simulink model "SimulateurNL_AERO_Cmd_LQI"  (R2023b)
settings: Solver=ode23tb  StartTime=0.0  StopTime=25  RelTol=1e-3
values from neighbouring files (symbols this model uses):
  Dm = 0.0071    [InitCommande_Aero.m]
  Dt = 0.158    [InitCommande_Aero.m]
  F0_h = Mb*g*Dm/Dt*sin(theta_h*pi/180)    [InitCommande_Aero.m]
  g = 9.81    [InitCommande_Aero.m]
  K_lqi = lqr(Aa, B1a, Q, R)    [InitCommande_Aero.m]
  Kw = Ka(1)    [InitCommande_Aero.m]    (also in matlab_variables_2_2.mat = 0.240350108962)
  Kz = Ka(2)    [InitCommande_Aero.m]    (also in matlab_variables_2_2.mat = 4.57892915652)
  Mb = 1.15    [InitCommande_Aero.m]
  omega_h = [-250 -200 -150 150 200 250]    [InitCommande_Aero.m]
  Te1 = 0.002    [InitCommande_Aero.m]    (also in apoio.m = 0.0005; matlab_variables_2_2.mat)
  Te2 = 0.02    [InitCommande_Aero.m]
libraries: simulink_extras x1
settings Model: Creator=Stagiaire  LastModifiedBy=rick
settings SolverCC: AlgebraicLoopSolver=TrustRegion
settings DataIOCC: ReturnWorkspaceOutputs=off
settings OptimizationCC: ReuseModelBlockBuffer=off
settings DebuggingCC: UnconnectedInputMsg=warning  UnconnectedOutputMsg=warning  UnconnectedLineMsg=warning  ArithmeticOperatorsInVariantConditions=warning
settings ModelReferenceCC: EnableRefExpFcnMdlSchedulingChecks=on
settings SFSimCC: CustomCodeUndefinedFunction=UseInterfaceOnly

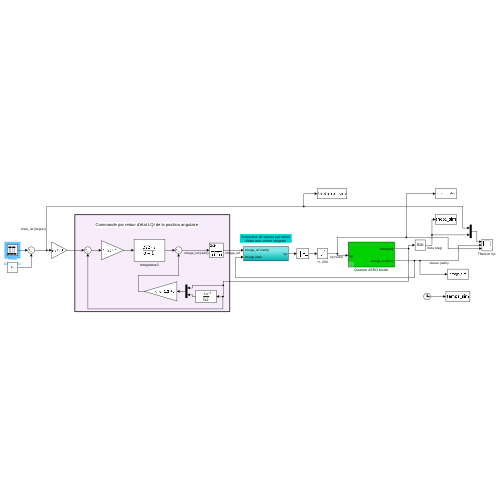
[thumbnail: Simulink's stored preview of the top-level diagram]
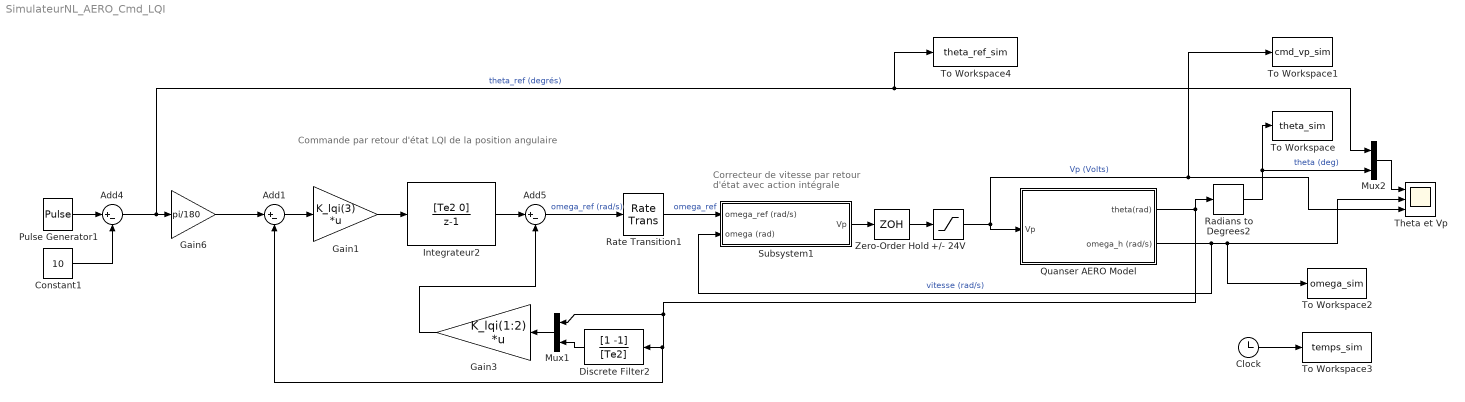
== system SimulateurNL_AERO_Cmd_LQI ==
  note: Correcteur de vitesse par retour d'état avec action intégrale
  note: Commande par retour d'état LQI de la position angulaire
  +/- 24V : Saturate  UpperLimit=24  LowerLimit=-24
  Add1 : Sum  Inputs=|+-
  Add4 : Sum  Inputs=|+-
  Add5 : Sum  Inputs=|+-
  Clock : Clock
  Constant1 : Constant  Value=10
  Discrete Filter2 : DiscreteFilter  Numerator=[1 -1]  Denominator=[Te2]  SampleTime=Te2
  Gain1 : Gain  Gain=K_lqi(3)  Multiplication=Matrix(K*u)
  Gain3 : Gain  Gain=K_lqi(1:2)  Multiplication=Matrix(K*u)
  Gain6 : Gain  Gain=pi/180
  Integrateur2 : DiscreteTransferFcn  Numerator=[Te2 0]  Denominator=[1 -1]  SampleTime=Te2
  Mux1 : Mux  Inputs=2
  Mux2 : Mux  Inputs=2
  Pulse Generator1 : DiscretePulseGenerator  Amplitude=20  Period=ceil(20/Te2)  PulseWidth=ceil(10/Te2)  SampleTime=Te2
  Quanser AERO Model : Subsystem  mask{Kv=19.66, tau=0.18, Jp=0.046, Dp=0.0091, F0_table=F0_h, W_table=omega_h}
  Radians to Degrees2 : simulink_extras/Transformations/Radians to Degrees
  Rate Transition1 : RateTransition  OutPortSampleTime=Te1
  Subsystem1 : Subsystem
  "Theta et Vp " : Scope  NumInputPorts=3
  To Workspace : ToWorkspace  VariableName=theta_sim  SampleTime=-1
      settings: Decimation=10  Save2DSignal=2-D array (concatenate along first dimension)
  To Workspace1 : ToWorkspace  VariableName=cmd_vp_sim  SampleTime=-1
      settings: Decimation=10  Save2DSignal=2-D array (concatenate along first dimension)
  To Workspace2 : ToWorkspace  VariableName=omega_sim  SampleTime=-1
      settings: Decimation=10  Save2DSignal=2-D array (concatenate along first dimension)
  To Workspace3 : ToWorkspace  VariableName=temps_sim  SampleTime=-1
      settings: Decimation=10  Save2DSignal=2-D array (concatenate along first dimension)
  To Workspace4 : ToWorkspace  VariableName=theta_ref_sim  SampleTime=-1
      settings: Decimation=10  Save2DSignal=2-D array (concatenate along first dimension)
  Zero-Order Hold : ZeroOrderHold  SampleTime=Te1
  wires:
  +/- 24V/1 -> To Workspace1/1, "Theta et Vp "/3, Quanser AERO Model/1(Vp)  "Vp (Volts)"
  Quanser AERO Model/2(omega_h (rad/s)) -> Subsystem1/2(omega (rad)), To Workspace2/1, "Theta et Vp "/2  "vitesse (rad/s)"
  Quanser AERO Model/1(theta(rad)) -> Radians to Degrees2/1, Add1/2, Discrete Filter2/1, Mux1/1
  Zero-Order Hold/1 -> +/- 24V/1
  Rate Transition1/1 -> Subsystem1/1(omega_ref (rad/s))  "omega_ref"
  Gain3/1 -> Add5/2
  Add5/1 -> Rate Transition1/1  "omega_ref (rad/s)"
  Mux1/1 -> Gain3/1
  Add4/1 -> To Workspace4/1, Mux2/1, Gain6/1  "theta_ref (degrés)"
  Pulse Generator1/1 -> Add4/1
  Constant1/1 -> Add4/2
  Subsystem1/1(Vp) -> Zero-Order Hold/1
  Mux2/1 -> "Theta et Vp "/1
  Radians to Degrees2/1 -> To Workspace/1, Mux2/2  "theta (deg)"
  Discrete Filter2/1 -> Mux1/2
  Gain1/1 -> Integrateur2/1
  Integrateur2/1 -> Add5/1
  Gain6/1 -> Add1/1
  Add1/1 -> Gain1/1
  Clock/1 -> To Workspace3/1

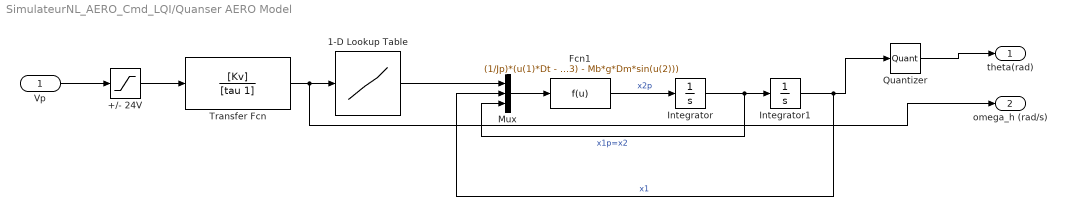
== system SimulateurNL_AERO_Cmd_LQI/Quanser AERO Model ==
  Vp : Inport
  +/- 24V : Saturate  UpperLimit=24  LowerLimit=-24
  1-D Lookup Table : Lookup_n-D  NumberOfTableDimensions=1  BreakpointsForDimension1=W_table  Table=F0_table  InternalRulePriority=Speed  RndMeth=Simplest
  Fcn1 : Fcn  Expr=(1/Jp)*(u(1)*Dt - Dp*u(3) - Mb*g*Dm*sin(u(2)))
  Integrator : Integrator
  Integrator1 : Integrator
  Mux : Mux  Inputs=3
  Quantizer : Quantizer  QuantizationInterval=2*pi/2048
  Transfer Fcn : TransferFcn  Numerator=[Kv]  Denominator=[tau 1]
  theta(rad) : Outport  VectorParamsAs1DForOutWhenUnconnected=off
  omega_h (rad/s) : Outport  Port=2  VectorParamsAs1DForOutWhenUnconnected=off
  wires:
  1-D Lookup Table/1 -> Mux/1
  Mux/1 -> Fcn1/1
  Integrator/1 -> Integrator1/1, Mux/3  "x1p=x2"
  Fcn1/1 -> Integrator/1  "x2p"
  Transfer Fcn/1 -> omega_h (rad/s)/1, 1-D Lookup Table/1
  Quantizer/1 -> theta(rad)/1
  Vp/1 -> +/- 24V/1
  Integrator1/1 -> Quantizer/1, Mux/2  "x1"
  +/- 24V/1 -> Transfer Fcn/1

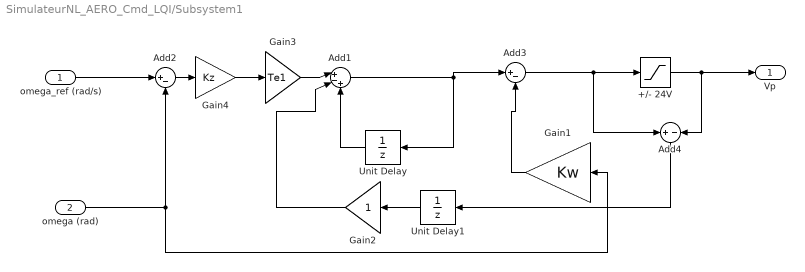
== system SimulateurNL_AERO_Cmd_LQI/Subsystem1 ==
  omega_ref (rad/s) : Inport
  omega (rad) : Inport  Port=2
  +/- 24V : Saturate  UpperLimit=24  LowerLimit=-24
  Add1 : Sum  Inputs=|+-+
  Add2 : Sum  Inputs=|+-
  Add3 : Sum  Inputs=|+-
  Add4 : Sum  Inputs=+-
  Gain1 : Gain  Gain=Kw
  Gain2 : Gain
  Gain3 : Gain  Gain=Te1
  Gain4 : Gain  Gain=Kz
  Unit Delay : UnitDelay  SampleTime=Te1  HasFrameUpgradeWarning=on
  Unit Delay1 : UnitDelay  SampleTime=Te1  HasFrameUpgradeWarning=on
  Vp : Outport  VectorParamsAs1DForOutWhenUnconnected=off
  wires:
  Gain2/1 -> Add1/2
  Gain1/1 -> Add3/2
  Add2/1 -> Gain4/1
  Add3/1 -> +/- 24V/1, Add4/1
  Unit Delay1/1 -> Gain2/1
  Gain4/1 -> Gain3/1
  Add4/1 -> Unit Delay1/1
  omega (rad)/1 -> Gain1/1, Add2/2
  omega_ref (rad/s)/1 -> Add2/1
  Gain3/1 -> Add1/1
  Add1/1 -> Add3/1, Unit Delay/1
  +/- 24V/1 -> Vp/1, Add4/2
  Unit Delay/1 -> Add1/3
